simulink subsystem "Server_sub"  (R2022b)
settings: Solver=VariableStepAuto  StartTime=0.0  StopTime=10.0  RelTol=1e-3
(part 2 of 2)

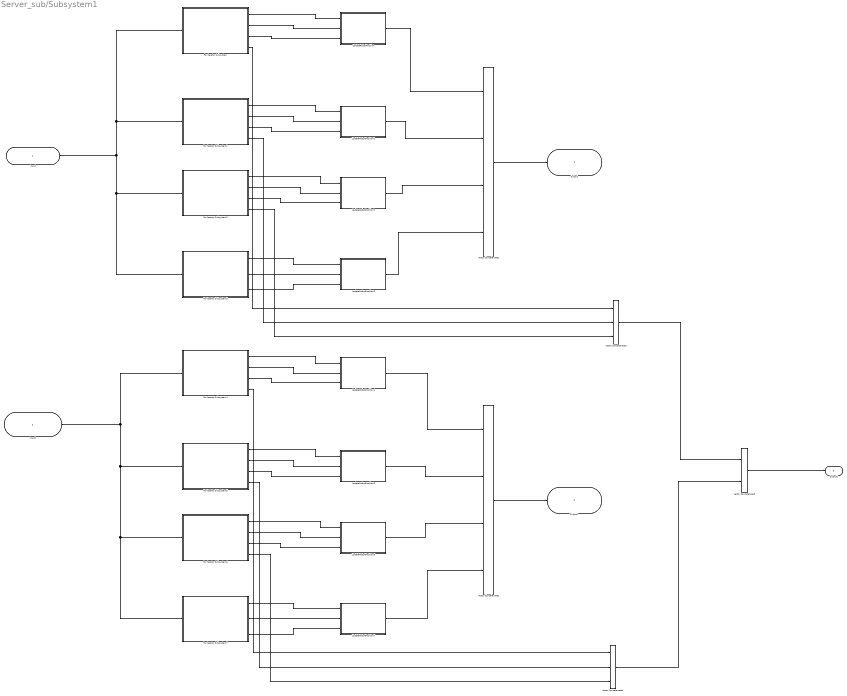
== system Server_sub/Subsystem1 ==
  Input : Inport
  Input1 : Inport  Port=2
  For Iterator Subsystem : Subsystem  TreatAsAtomicUnit=on
  For Iterator Subsystem1 : Subsystem  TreatAsAtomicUnit=on
  For Iterator Subsystem2 : Subsystem  TreatAsAtomicUnit=on
  For Iterator Subsystem3 : Subsystem  TreatAsAtomicUnit=on
  For Iterator Subsystem4 : Subsystem  TreatAsAtomicUnit=on
  For Iterator Subsystem5 : Subsystem  TreatAsAtomicUnit=on
  For Iterator Subsystem6 : Subsystem  TreatAsAtomicUnit=on
  For Iterator Subsystem7 : Subsystem  TreatAsAtomicUnit=on
  UpdateRobotPosition : MATLAB Function  TreatAsAtomicUnit=on
  UpdateRobotPosition1 : MATLAB Function  TreatAsAtomicUnit=on
  UpdateRobotPosition2 : MATLAB Function  TreatAsAtomicUnit=on
  UpdateRobotPosition3 : MATLAB Function  TreatAsAtomicUnit=on
  UpdateRobotPosition4 : MATLAB Function  TreatAsAtomicUnit=on
  UpdateRobotPosition5 : MATLAB Function  TreatAsAtomicUnit=on
  UpdateRobotPosition6 : MATLAB Function  TreatAsAtomicUnit=on
  UpdateRobotPosition7 : MATLAB Function  TreatAsAtomicUnit=on
  Vector Concatenate1 : Concatenate  NumInputs=4  Mode=Multidimensional array
  Vector Concatenate2 : Concatenate  NumInputs=4  Mode=Multidimensional array
  Vector Concatenate3 : Concatenate  NumInputs=3  Mode=Multidimensional array
  Vector Concatenate4 : Concatenate  NumInputs=3  Mode=Multidimensional array
  Vector Concatenate5 : Concatenate  Mode=Multidimensional array
  Output : Outport
  Output1 : Outport  Port=2
  Output2 : Outport  Port=3
  wires:
  For Iterator Subsystem2/4(kick) -> Vector Concatenate3/3
  Vector Concatenate5/1 -> Output2/1
  Vector Concatenate4/1 -> Vector Concatenate5/2
  Vector Concatenate3/1 -> Vector Concatenate5/1
  For Iterator Subsystem/4(kick) -> Vector Concatenate3/1
  For Iterator Subsystem1/4(kick) -> Vector Concatenate3/2
  For Iterator Subsystem6/4(kick) -> Vector Concatenate4/3
  For Iterator Subsystem5/4(kick) -> Vector Concatenate4/2
  For Iterator Subsystem4/4(kick) -> Vector Concatenate4/1
  For Iterator Subsystem1/3(heading1) -> UpdateRobotPosition1/3(heading1)
  For Iterator Subsystem1/1(x) -> UpdateRobotPosition1/1(currentX1)
  UpdateRobotPosition4/1(robot_coordinates5) -> Vector Concatenate2/1
  UpdateRobotPosition5/1(robot_coordinates6) -> Vector Concatenate2/2
  UpdateRobotPosition/1(robot_coordinates1) -> Vector Concatenate1/1
  UpdateRobotPosition3/1(robot_coordinates4) -> Vector Concatenate1/4
  For Iterator Subsystem5/2(y) -> UpdateRobotPosition5/2(currentY1)
  For Iterator Subsystem6/1(x) -> UpdateRobotPosition6/1(currentX1)
  For Iterator Subsystem5/3(heading1) -> UpdateRobotPosition5/3(heading1)
  For Iterator Subsystem4/2(y) -> UpdateRobotPosition4/2(currentY1)
  For Iterator Subsystem4/3(heading1) -> UpdateRobotPosition4/3(heading1)
  For Iterator Subsystem6/3(heading1) -> UpdateRobotPosition6/3(heading1)
  For Iterator Subsystem6/2(y) -> UpdateRobotPosition6/2(currentY1)
  For Iterator Subsystem1/2(y) -> UpdateRobotPosition1/2(currentY1)
  For Iterator Subsystem4/1(x) -> UpdateRobotPosition4/1(currentX1)
  For Iterator Subsystem7/3(heading1) -> UpdateRobotPosition7/3(heading1)
  For Iterator Subsystem7/1(x) -> UpdateRobotPosition7/1(currentX1)
  For Iterator Subsystem5/1(x) -> UpdateRobotPosition5/1(currentX1)
  For Iterator Subsystem7/2(y) -> UpdateRobotPosition7/2(currentY1)
  For Iterator Subsystem3/1(x) -> UpdateRobotPosition3/1(currentX1)
  For Iterator Subsystem3/3(heading1) -> UpdateRobotPosition3/3(heading1)
  For Iterator Subsystem/1(x) -> UpdateRobotPosition/1(currentX1)
  For Iterator Subsystem2/3(heading1) -> UpdateRobotPosition2/3(heading1)
  UpdateRobotPosition1/1(robot_coordinates2) -> Vector Concatenate1/2
  UpdateRobotPosition2/1(robot_coordinates3) -> Vector Concatenate1/3
  For Iterator Subsystem2/2(y) -> UpdateRobotPosition2/2(currentY1)
  For Iterator Subsystem/2(y) -> UpdateRobotPosition/2(currentY1)
  For Iterator Subsystem2/1(x) -> UpdateRobotPosition2/1(currentX1)
  UpdateRobotPosition7/1(robot_coordinates8) -> Vector Concatenate2/4
  For Iterator Subsystem/3(heading1) -> UpdateRobotPosition/3(heading1)
  For Iterator Subsystem3/2(y) -> UpdateRobotPosition3/2(currentY1)
  UpdateRobotPosition6/1(robot_coordinates7) -> Vector Concatenate2/3
  Vector Concatenate1/1 -> Output/1
  Input/1 -> For Iterator Subsystem3/1(robot), For Iterator Subsystem2/1(robot), For Iterator Subsystem1/1(robot), For Iterator Subsystem/1(robot)
  Input1/1 -> For Iterator Subsystem4/1(robot), For Iterator Subsystem5/1(robot), For Iterator Subsystem7/1(robot), For Iterator Subsystem6/1(robot)
  Vector Concatenate2/1 -> Output1/1

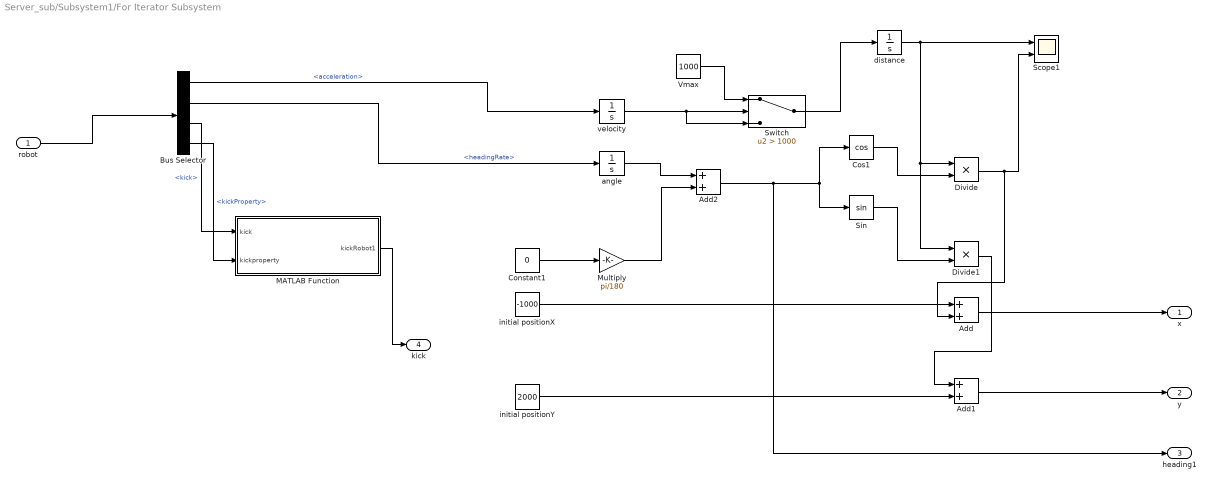
== system Server_sub/Subsystem1/For Iterator Subsystem ==
  robot : Inport
  Add : Sum
  Add1 : Sum
  Add2 : Sum
  Bus Selector : BusSelector  OutputSignals=signal1.acceleration,signal1.headingRate,signal1.kick,signal1.kickProperty
  Constant1 : Constant  Value=0
  Cos1 : Trigonometry  Operator=cos
  Divide : Product  Inputs=**
  Divide1 : Product  Inputs=**
  MATLAB Function : MATLAB Function  TreatAsAtomicUnit=on
  Multiply : Gain  Gain=pi/180
  Scope1 : Scope  NumInputPorts=2
  Sin : Trigonometry
  Switch : Switch  Criteria=u2 > Threshold  Threshold=1000  SaturateOnIntegerOverflow=off  InputSameDT=off
  "Vmax " : Constant  Value=1000
  angle : Integrator
  distance : Integrator
  initial positionX : Constant  Value=-1000
  initial positionY : Constant  Value=2000
  velocity : Integrator
  x : Outport
  y : Outport  Port=2
  heading1 : Outport  Port=3
  kick : Outport  Port=4
  wires:
  MATLAB Function/1(kickRobot1) -> kick/1
  Bus Selector/4 -> MATLAB Function/2(kickproperty)  "<kickProperty>"
  Bus Selector/3 -> MATLAB Function/1(kick)  "<kick>"
  initial positionX/1 -> Add/1
  initial positionY/1 -> Add1/2
  Sin/1 -> Divide1/2
  distance/1 -> Divide1/1, Divide/1, Scope1/1
  Cos1/1 -> Divide/2
  Divide/1 -> Add/2, Scope1/2
  "Vmax "/1 -> Switch/1
  Switch/1 -> distance/1
  velocity/1 -> Switch/3, Switch/2
  Add/1 -> x/1
  Divide1/1 -> Add1/1
  Add1/1 -> y/1
  angle/1 -> Add2/1
  Constant1/1 -> Multiply/1
  Add2/1 -> heading1/1, Cos1/1, Sin/1
  Multiply/1 -> Add2/2
  robot/1 -> Bus Selector/1
  Bus Selector/1 -> velocity/1  "<acceleration>"
  Bus Selector/2 -> angle/1  "<headingRate>"

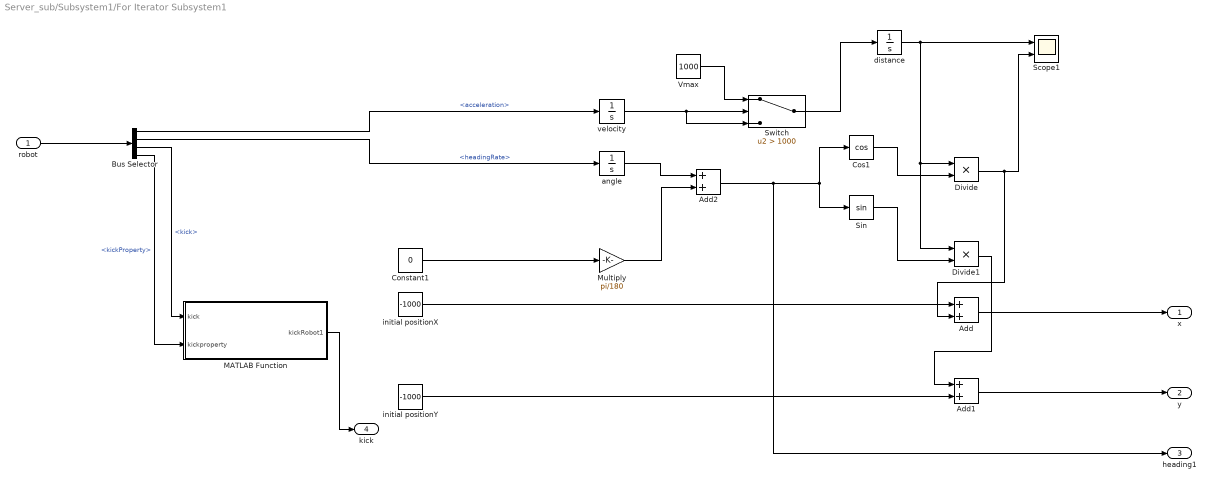
== system Server_sub/Subsystem1/For Iterator Subsystem1 ==
  robot : Inport
  Add : Sum
  Add1 : Sum
  Add2 : Sum
  Bus Selector : BusSelector  OutputSignals=signal2.acceleration,signal2.headingRate,signal2.kick,signal2.kickProperty
  Constant1 : Constant  Value=0
  Cos1 : Trigonometry  Operator=cos
  Divide : Product  Inputs=**
  Divide1 : Product  Inputs=**
  MATLAB Function : MATLAB Function  TreatAsAtomicUnit=on
  Multiply : Gain  Gain=pi/180
  Scope1 : Scope  NumInputPorts=2
  Sin : Trigonometry
  Switch : Switch  Criteria=u2 > Threshold  Threshold=1000  SaturateOnIntegerOverflow=off  InputSameDT=off
  "Vmax " : Constant  Value=1000
  angle : Integrator
  distance : Integrator
  initial positionX : Constant  Value=-1000
  initial positionY : Constant  Value=-1000
  velocity : Integrator
  x : Outport
  y : Outport  Port=2
  heading1 : Outport  Port=3
  kick : Outport  Port=4
  wires:
  Bus Selector/4 -> MATLAB Function/2(kickproperty)  "<kickProperty>"
  Bus Selector/3 -> MATLAB Function/1(kick)  "<kick>"
  MATLAB Function/1(kickRobot1) -> kick/1
  initial positionX/1 -> Add/1
  initial positionY/1 -> Add1/2
  Sin/1 -> Divide1/2
  distance/1 -> Divide1/1, Divide/1, Scope1/1
  Cos1/1 -> Divide/2
  Divide/1 -> Add/2, Scope1/2
  "Vmax "/1 -> Switch/1
  Switch/1 -> distance/1
  velocity/1 -> Switch/3, Switch/2
  Add/1 -> x/1
  Divide1/1 -> Add1/1
  Add1/1 -> y/1
  angle/1 -> Add2/1
  Constant1/1 -> Multiply/1
  Add2/1 -> heading1/1, Cos1/1, Sin/1
  Multiply/1 -> Add2/2
  robot/1 -> Bus Selector/1
  Bus Selector/1 -> velocity/1  "<acceleration>"
  Bus Selector/2 -> angle/1  "<headingRate>"

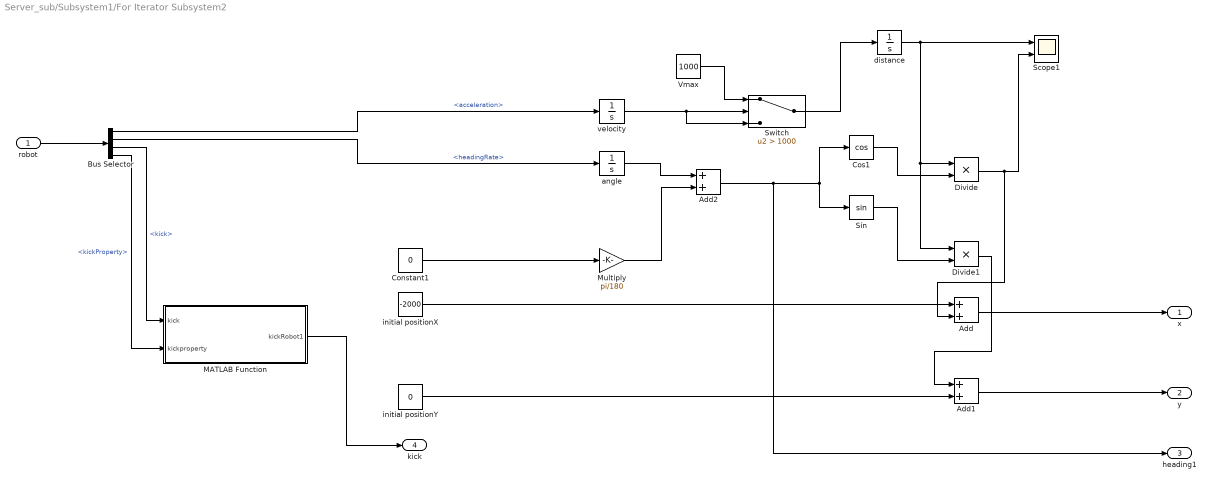
== system Server_sub/Subsystem1/For Iterator Subsystem2 ==
  robot : Inport
  Add : Sum
  Add1 : Sum
  Add2 : Sum
  Bus Selector : BusSelector  OutputSignals=signal3.acceleration,signal3.headingRate,signal3.kick,signal3.kickProperty
  Constant1 : Constant  Value=0
  Cos1 : Trigonometry  Operator=cos
  Divide : Product  Inputs=**
  Divide1 : Product  Inputs=**
  MATLAB Function : MATLAB Function  TreatAsAtomicUnit=on
  Multiply : Gain  Gain=pi/180
  Scope1 : Scope  NumInputPorts=2
  Sin : Trigonometry
  Switch : Switch  Criteria=u2 > Threshold  Threshold=1000  SaturateOnIntegerOverflow=off  InputSameDT=off
  "Vmax " : Constant  Value=1000
  angle : Integrator
  distance : Integrator
  initial positionX : Constant  Value=-2000
  initial positionY : Constant  Value=0
  velocity : Integrator
  x : Outport
  y : Outport  Port=2
  heading1 : Outport  Port=3
  kick : Outport  Port=4
  wires:
  Bus Selector/4 -> MATLAB Function/2(kickproperty)  "<kickProperty>"
  Bus Selector/3 -> MATLAB Function/1(kick)  "<kick>"
  MATLAB Function/1(kickRobot1) -> kick/1
  initial positionX/1 -> Add/1
  initial positionY/1 -> Add1/2
  Sin/1 -> Divide1/2
  distance/1 -> Divide1/1, Divide/1, Scope1/1
  Cos1/1 -> Divide/2
  Divide/1 -> Add/2, Scope1/2
  "Vmax "/1 -> Switch/1
  Switch/1 -> distance/1
  velocity/1 -> Switch/3, Switch/2
  Add/1 -> x/1
  Divide1/1 -> Add1/1
  Add1/1 -> y/1
  angle/1 -> Add2/1
  Constant1/1 -> Multiply/1
  Add2/1 -> heading1/1, Cos1/1, Sin/1
  Multiply/1 -> Add2/2
  robot/1 -> Bus Selector/1
  Bus Selector/1 -> velocity/1  "<acceleration>"
  Bus Selector/2 -> angle/1  "<headingRate>"

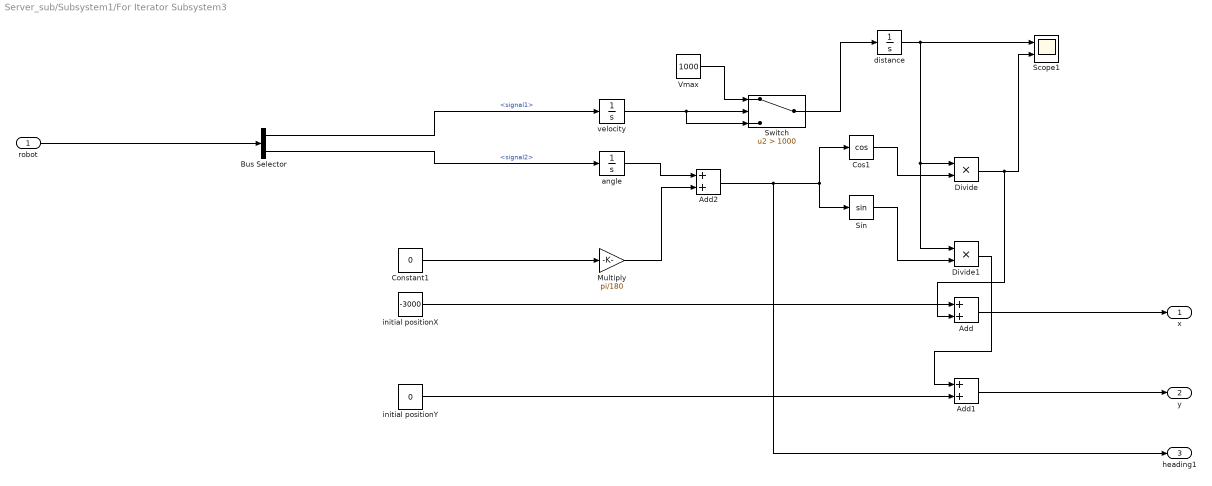
== system Server_sub/Subsystem1/For Iterator Subsystem3 ==
  robot : Inport
  Add : Sum
  Add1 : Sum
  Add2 : Sum
  Bus Selector : BusSelector  OutputSignals=signal1,signal2
  Constant1 : Constant  Value=0
  Cos1 : Trigonometry  Operator=cos
  Divide : Product  Inputs=**
  Divide1 : Product  Inputs=**
  Multiply : Gain  Gain=pi/180
  Scope1 : Scope  NumInputPorts=2
  Sin : Trigonometry
  Switch : Switch  Criteria=u2 > Threshold  Threshold=1000  SaturateOnIntegerOverflow=off  InputSameDT=off
  "Vmax " : Constant  Value=1000
  angle : Integrator
  distance : Integrator
  initial positionX : Constant  Value=-3000
  initial positionY : Constant  Value=0
  velocity : Integrator
  x : Outport
  y : Outport  Port=2
  heading1 : Outport  Port=3
  wires:
  initial positionX/1 -> Add/1
  initial positionY/1 -> Add1/2
  Sin/1 -> Divide1/2
  distance/1 -> Divide1/1, Divide/1, Scope1/1
  Cos1/1 -> Divide/2
  Divide/1 -> Add/2, Scope1/2
  "Vmax "/1 -> Switch/1
  Switch/1 -> distance/1
  velocity/1 -> Switch/3, Switch/2
  Add/1 -> x/1
  Divide1/1 -> Add1/1
  Add1/1 -> y/1
  angle/1 -> Add2/1
  Constant1/1 -> Multiply/1
  Add2/1 -> heading1/1, Cos1/1, Sin/1
  Multiply/1 -> Add2/2
  robot/1 -> Bus Selector/1
  Bus Selector/1 -> velocity/1  "<signal1>"
  Bus Selector/2 -> angle/1  "<signal2>"

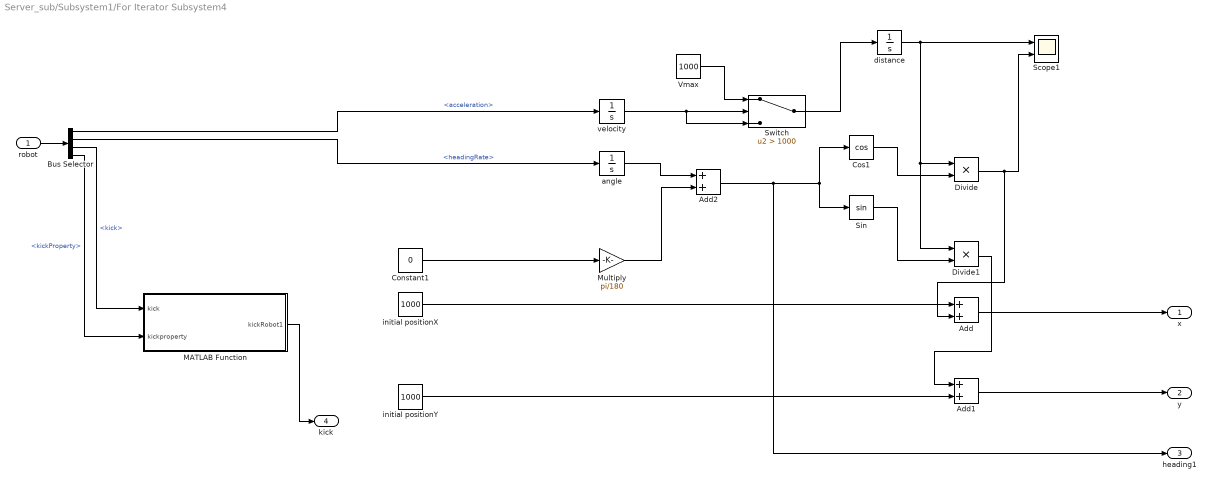
== system Server_sub/Subsystem1/For Iterator Subsystem4 ==
  robot : Inport
  Add : Sum
  Add1 : Sum
  Add2 : Sum
  Bus Selector : BusSelector  OutputSignals=signal1.acceleration,signal1.headingRate,signal1.kick,signal1.kickProperty
  Constant1 : Constant  Value=0
  Cos1 : Trigonometry  Operator=cos
  Divide : Product  Inputs=**
  Divide1 : Product  Inputs=**
  MATLAB Function : MATLAB Function  TreatAsAtomicUnit=on
  Multiply : Gain  Gain=pi/180
  Scope1 : Scope  NumInputPorts=2
  Sin : Trigonometry
  Switch : Switch  Criteria=u2 > Threshold  Threshold=1000  SaturateOnIntegerOverflow=off  InputSameDT=off
  "Vmax " : Constant  Value=1000
  angle : Integrator
  distance : Integrator
  initial positionX : Constant  Value=1000
  initial positionY : Constant  Value=1000
  velocity : Integrator
  x : Outport
  y : Outport  Port=2
  heading1 : Outport  Port=3
  kick : Outport  Port=4
  wires:
  Bus Selector/4 -> MATLAB Function/2(kickproperty)  "<kickProperty>"
  Bus Selector/3 -> MATLAB Function/1(kick)  "<kick>"
  MATLAB Function/1(kickRobot1) -> kick/1
  initial positionX/1 -> Add/1
  initial positionY/1 -> Add1/2
  Sin/1 -> Divide1/2
  distance/1 -> Divide1/1, Divide/1, Scope1/1
  Cos1/1 -> Divide/2
  Divide/1 -> Add/2, Scope1/2
  "Vmax "/1 -> Switch/1
  Switch/1 -> distance/1
  velocity/1 -> Switch/3, Switch/2
  Add/1 -> x/1
  Divide1/1 -> Add1/1
  Add1/1 -> y/1
  angle/1 -> Add2/1
  Constant1/1 -> Multiply/1
  Add2/1 -> heading1/1, Cos1/1, Sin/1
  Multiply/1 -> Add2/2
  robot/1 -> Bus Selector/1
  Bus Selector/1 -> velocity/1  "<acceleration>"
  Bus Selector/2 -> angle/1  "<headingRate>"

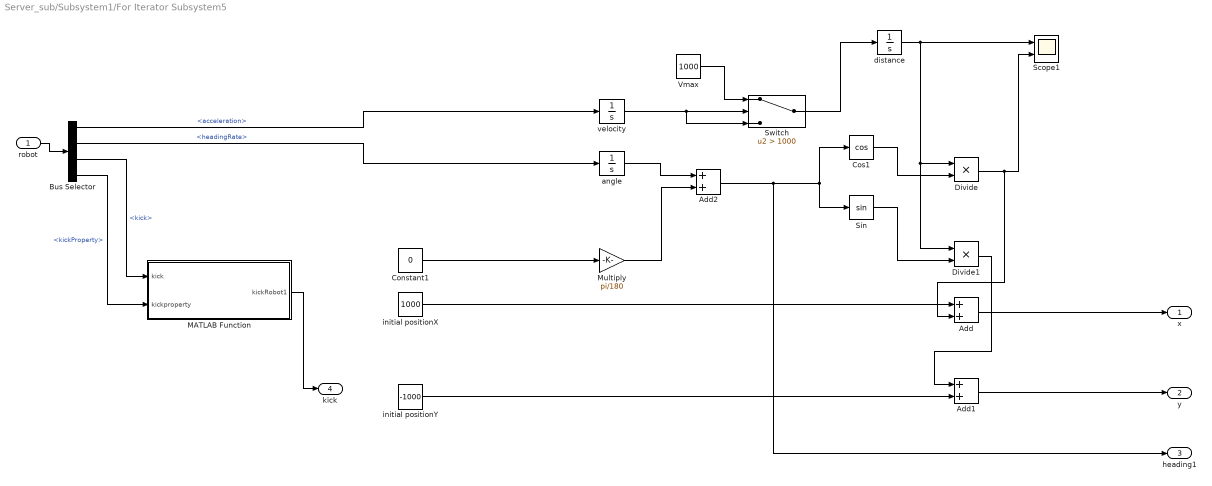
== system Server_sub/Subsystem1/For Iterator Subsystem5 ==
  robot : Inport
  Add : Sum
  Add1 : Sum
  Add2 : Sum
  Bus Selector : BusSelector  OutputSignals=signal2.acceleration,signal2.headingRate,signal2.kick,signal2.kickProperty
  Constant1 : Constant  Value=0
  Cos1 : Trigonometry  Operator=cos
  Divide : Product  Inputs=**
  Divide1 : Product  Inputs=**
  MATLAB Function : MATLAB Function  TreatAsAtomicUnit=on
  Multiply : Gain  Gain=pi/180
  Scope1 : Scope  NumInputPorts=2
  Sin : Trigonometry
  Switch : Switch  Criteria=u2 > Threshold  Threshold=1000  SaturateOnIntegerOverflow=off  InputSameDT=off
  "Vmax " : Constant  Value=1000
  angle : Integrator
  distance : Integrator
  initial positionX : Constant  Value=1000
  initial positionY : Constant  Value=-1000
  velocity : Integrator
  x : Outport
  y : Outport  Port=2
  heading1 : Outport  Port=3
  kick : Outport  Port=4
  wires:
  Bus Selector/4 -> MATLAB Function/2(kickproperty)  "<kickProperty>"
  Bus Selector/3 -> MATLAB Function/1(kick)  "<kick>"
  MATLAB Function/1(kickRobot1) -> kick/1
  initial positionX/1 -> Add/1
  initial positionY/1 -> Add1/2
  Sin/1 -> Divide1/2
  distance/1 -> Divide1/1, Divide/1, Scope1/1
  Cos1/1 -> Divide/2
  Divide/1 -> Add/2, Scope1/2
  "Vmax "/1 -> Switch/1
  Switch/1 -> distance/1
  velocity/1 -> Switch/3, Switch/2
  Add/1 -> x/1
  Divide1/1 -> Add1/1
  Add1/1 -> y/1
  angle/1 -> Add2/1
  Constant1/1 -> Multiply/1
  Add2/1 -> heading1/1, Cos1/1, Sin/1
  Multiply/1 -> Add2/2
  robot/1 -> Bus Selector/1
  Bus Selector/1 -> velocity/1  "<acceleration>"
  Bus Selector/2 -> angle/1  "<headingRate>"

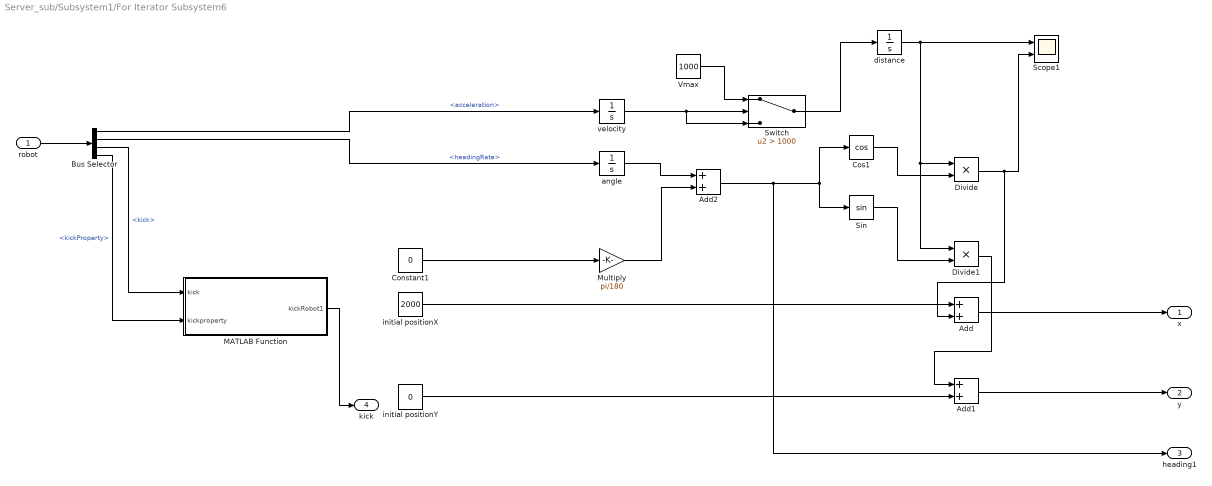
== system Server_sub/Subsystem1/For Iterator Subsystem6 ==
  robot : Inport
  Add : Sum
  Add1 : Sum
  Add2 : Sum
  Bus Selector : BusSelector  OutputSignals=signal3.acceleration,signal3.headingRate,signal3.kick,signal3.kickProperty
  Constant1 : Constant  Value=0
  Cos1 : Trigonometry  Operator=cos
  Divide : Product  Inputs=**
  Divide1 : Product  Inputs=**
  MATLAB Function : MATLAB Function  TreatAsAtomicUnit=on
  Multiply : Gain  Gain=pi/180
  Scope1 : Scope  NumInputPorts=2
  Sin : Trigonometry
  Switch : Switch  Criteria=u2 > Threshold  Threshold=1000  SaturateOnIntegerOverflow=off  InputSameDT=off
  "Vmax " : Constant  Value=1000
  angle : Integrator
  distance : Integrator
  initial positionX : Constant  Value=2000
  initial positionY : Constant  Value=0
  velocity : Integrator
  x : Outport
  y : Outport  Port=2
  heading1 : Outport  Port=3
  kick : Outport  Port=4
  wires:
  Bus Selector/4 -> MATLAB Function/2(kickproperty)  "<kickProperty>"
  Bus Selector/3 -> MATLAB Function/1(kick)  "<kick>"
  MATLAB Function/1(kickRobot1) -> kick/1
  initial positionX/1 -> Add/1
  initial positionY/1 -> Add1/2
  Sin/1 -> Divide1/2
  distance/1 -> Divide1/1, Divide/1, Scope1/1
  Cos1/1 -> Divide/2
  Divide/1 -> Add/2, Scope1/2
  "Vmax "/1 -> Switch/1
  Switch/1 -> distance/1
  velocity/1 -> Switch/3, Switch/2
  Add/1 -> x/1
  Divide1/1 -> Add1/1
  Add1/1 -> y/1
  angle/1 -> Add2/1
  Constant1/1 -> Multiply/1
  Add2/1 -> heading1/1, Cos1/1, Sin/1
  Multiply/1 -> Add2/2
  robot/1 -> Bus Selector/1
  Bus Selector/1 -> velocity/1  "<acceleration>"
  Bus Selector/2 -> angle/1  "<headingRate>"

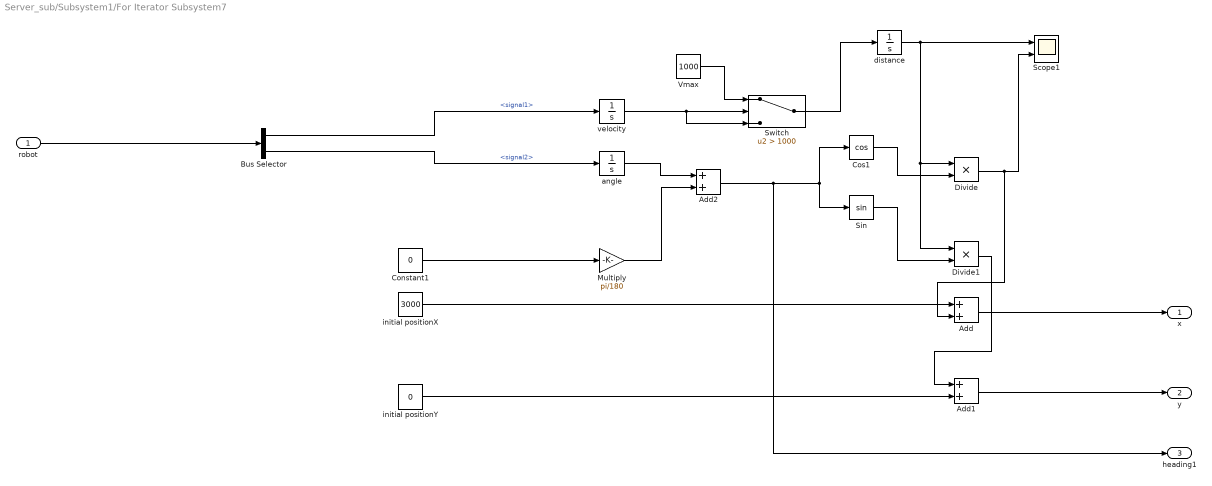
== system Server_sub/Subsystem1/For Iterator Subsystem7 ==
  robot : Inport
  Add : Sum
  Add1 : Sum
  Add2 : Sum
  Bus Selector : BusSelector  OutputSignals=signal1,signal2
  Constant1 : Constant  Value=0
  Cos1 : Trigonometry  Operator=cos
  Divide : Product  Inputs=**
  Divide1 : Product  Inputs=**
  Multiply : Gain  Gain=pi/180
  Scope1 : Scope  NumInputPorts=2
  Sin : Trigonometry
  Switch : Switch  Criteria=u2 > Threshold  Threshold=1000  SaturateOnIntegerOverflow=off  InputSameDT=off
  "Vmax " : Constant  Value=1000
  angle : Integrator
  distance : Integrator
  initial positionX : Constant  Value=3000
  initial positionY : Constant  Value=0
  velocity : Integrator
  x : Outport
  y : Outport  Port=2
  heading1 : Outport  Port=3
  wires:
  initial positionX/1 -> Add/1
  initial positionY/1 -> Add1/2
  Sin/1 -> Divide1/2
  distance/1 -> Divide1/1, Divide/1, Scope1/1
  Cos1/1 -> Divide/2
  Divide/1 -> Add/2, Scope1/2
  "Vmax "/1 -> Switch/1
  Switch/1 -> distance/1
  velocity/1 -> Switch/3, Switch/2
  Add/1 -> x/1
  Divide1/1 -> Add1/1
  Add1/1 -> y/1
  angle/1 -> Add2/1
  Constant1/1 -> Multiply/1
  Add2/1 -> heading1/1, Cos1/1, Sin/1
  Multiply/1 -> Add2/2
  robot/1 -> Bus Selector/1
  Bus Selector/1 -> velocity/1  "<signal1>"
  Bus Selector/2 -> angle/1  "<signal2>"

== matlab function Server_sub/Subsystem1/UpdateRobotPosition2 ==
  data: currentX1 input; robot_coordinates3 output; currentY1 input; heading1 input
function robot_coordinates3  = UpdateRobotPosition(currentX1, currentY1, heading1)

 
    % put heading in vector
    currentPosition = [currentX1, currentY1, heading1];
    
   
    % output the vector
    robot_coordinates3 = currentPosition;
end

== matlab function Server_sub/Subsystem1/UpdateRobotPosition3 ==
  data: currentX1 input; robot_coordinates4 output; currentY1 input; heading1 input
function robot_coordinates4  = UpdateRobotPosition(currentX1, currentY1, heading1)

 
    % put heading in vector
    currentPosition = [currentX1, currentY1, heading1];
    
   
    % output the vector
    robot_coordinates4 = currentPosition;
end

== matlab function Server_sub/Subsystem1/UpdateRobotPosition4 ==
  data: currentX1 input; robot_coordinates5 output; currentY1 input; heading1 input
function robot_coordinates5 = UpdateRobotPosition(currentX1, currentY1, heading1)

 
    % put heading in vector
    currentPosition = [currentX1, currentY1, heading1];
    
   
    % output the vector
    robot_coordinates5 = currentPosition;
end

== matlab function Server_sub/Subsystem1/UpdateRobotPosition5 ==
  data: currentX1 input; robot_coordinates6 output; currentY1 input; heading1 input
function robot_coordinates6  = UpdateRobotPosition(currentX1, currentY1, heading1)

 
    % put heading in vector
    currentPosition = [currentX1, currentY1, heading1];
    
   
    % output the vector
    robot_coordinates6 = currentPosition;
end

== matlab function Server_sub/Subsystem1/UpdateRobotPosition6 ==
  data: currentX1 input; robot_coordinates7 output; currentY1 input; heading1 input
function robot_coordinates7  = UpdateRobotPosition(currentX1, currentY1, heading1)

 
    % put heading in vector
    currentPosition = [currentX1, currentY1, heading1];
    
   
    % output the vector
    robot_coordinates7 = currentPosition;
end

== matlab function Server_sub/Subsystem1/UpdateRobotPosition7 ==
  data: currentX1 input; robot_coordinates8 output; currentY1 input; heading1 input
function robot_coordinates8  = UpdateRobotPosition(currentX1, currentY1, heading1)

 
    % put heading in vector
    currentPosition = [currentX1, currentY1, heading1];
    
   
    % output the vector
    robot_coordinates8 = currentPosition;
end

== matlab function Server_sub/MATLAB Function2 ==
  data: kickAndProperties input; kick output; kickProperties output
function [kick, kickProperties] = fcn(kickAndProperties)

kick = kickAndProperties(:,1);
kickProperties = kickAndProperties(:,2);

== matlab function Server_sub/MATLAB Function ==
  data: u input; y output
function y = foulSignal(u)
% Add logic to pause game and start penalty/free kick
y = u;

== matlab function Server_sub/MATLAB Function1 ==
  data: u input; y output
function y = offsideSignal(u)
% Add logic to pause game and start penalty/free kick
y = u;

== matlab function Server_sub/Subsystem1/For Iterator Subsystem/MATLAB Function ==
  data: kick input; kickRobot1 output; kickproperty input
function kickRobot1= kickCombine(kick,kickproperty)

 
    % put heading in vector
    kickRobot1 = [kick, kickproperty];
   
end

== matlab function Server_sub/Subsystem1/For Iterator Subsystem1/MATLAB Function ==
  data: kick input; kickRobot1 output; kickproperty input
function kickRobot1= kickCombine(kick,kickproperty)

 
    % put heading in vector
    kickRobot1 = [kick, kickproperty];
   
end

== matlab function Server_sub/Subsystem1/For Iterator Subsystem2/MATLAB Function ==
  data: kick input; kickRobot1 output; kickproperty input
function kickRobot1= kickCombine(kick,kickproperty)

 
    % put heading in vector
    kickRobot1 = [kick, kickproperty];
   
end

== matlab function Server_sub/Subsystem1/For Iterator Subsystem4/MATLAB Function ==
  data: kick input; kickRobot1 output; kickproperty input
function kickRobot1= kickCombine(kick,kickproperty)

 
    % put heading in vector
    kickRobot1 = [kick, kickproperty];
   
end

== matlab function Server_sub/Subsystem1/For Iterator Subsystem5/MATLAB Function ==
  data: kick input; kickRobot1 output; kickproperty input
function kickRobot1= kickCombine(kick,kickproperty)

 
    % put heading in vector
    kickRobot1 = [kick, kickproperty];
   
end

== matlab function Server_sub/Subsystem1/For Iterator Subsystem6/MATLAB Function ==
  data: kick input; kickRobot1 output; kickproperty input
function kickRobot1= kickCombine(kick,kickproperty)

 
    % put heading in vector
    kickRobot1 = [kick, kickproperty];
   
end

== matlab function Server_sub/Subsystem1/UpdateRobotPosition ==
  data: currentX1 input; robot_coordinates1 output; currentY1 input; heading1 input
function robot_coordinates1  = UpdateRobotPosition(currentX1, currentY1, heading1)

 
    % put heading in vector
    currentPosition = [currentX1, currentY1, heading1];
    
   
    % output the vector
    robot_coordinates1 = currentPosition;
end

== matlab function Server_sub/Subsystem1/UpdateRobotPosition1 ==
  data: currentX1 input; robot_coordinates2 output; currentY1 input; heading1 input
function robot_coordinates2  = UpdateRobotPosition(currentX1, currentY1, heading1)

 
    % put heading in vector
    currentPosition = [currentX1, currentY1, heading1];
    
   
    % output the vector
    robot_coordinates2 = currentPosition;
end
